simulink model "MatlabFunctionBlock"  (R2016a)
settings: Solver=VariableStepAuto  StartTime=0.0  StopTime=10  RelTol=1e-3
settings Model: Creator=DELL  LastModifiedBy=DELL

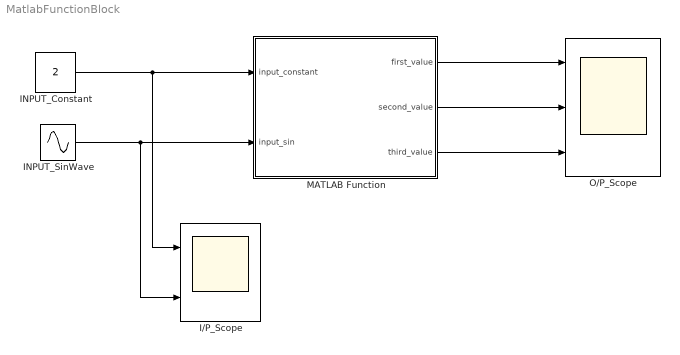
== system MatlabFunctionBlock ==
  I/P_Scope : Scope  NumInputPorts=2
  INPUT_Constant : Constant  Value=2
  INPUT_SinWave : Sin  Amplitude=5  SampleTime=0
  MATLAB Function : MATLAB Function  TreatAsAtomicUnit=on
  O/P_Scope : Scope  NumInputPorts=3
  wires:
  INPUT_Constant/1 -> I/P_Scope/1, MATLAB Function/1(input_constant)
  MATLAB Function/1(first_value) -> O/P_Scope/1
  INPUT_SinWave/1 -> I/P_Scope/2, MATLAB Function/2(input_sin)
  MATLAB Function/2(second_value) -> O/P_Scope/2
  MATLAB Function/3(third_value) -> O/P_Scope/3

== matlab function MatlabFunctionBlock/MATLAB Function ==
  data: input_constant input; first_value output; input_sin input; second_value output; third_value output
function [first_value,second_value,third_value] = my_Func(input_constant,input_sin)
%#codegen
first_value = input_sin + input_constant;
second_value = input_sin * input_constant;
third_value = first_value - input_sin;
end
